simulink model "gm_FCS_MPC_3Phase_SPMSM_V1"  (R2022a)
settings: Solver=ode23t  StartTime=0.0  StopTime=0.2  RelTol=1e-3  AbsTol=1e-3  EnableMultiTasking=on
undefined symbols (not defined in the file or in its folder): f_c, Ld, Lq, np, psiPM, R, T_50MHz, u_dc
libraries: hdlmdlgenlib x28, dspsigops x26, ee_lib x22, nesl_utility x22, fl_lib x21, simulink x7
(part 2 of 5)

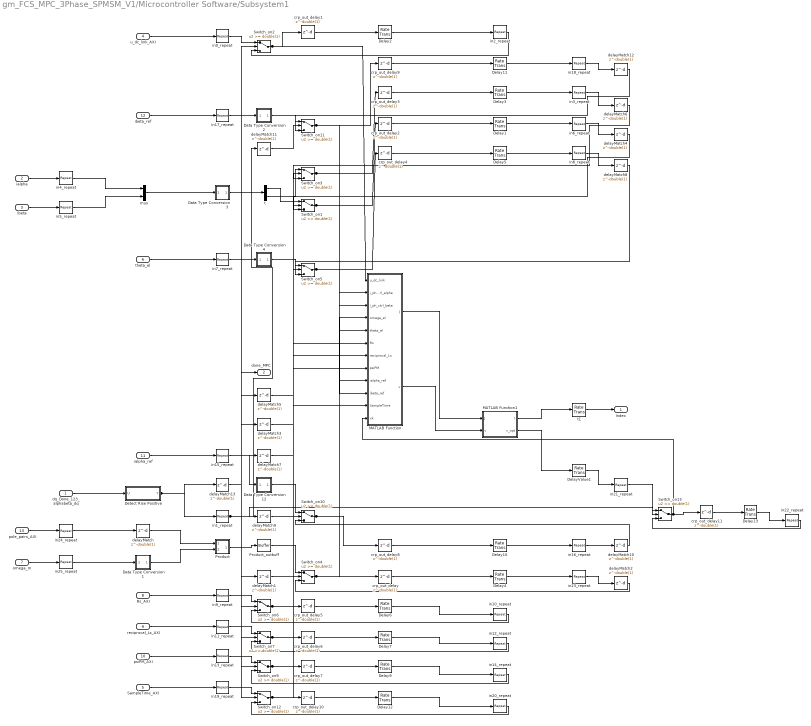
== system gm_FCS_MPC_3Phase_SPMSM_V1/Microcontroller Software/Subsystem1 ==
  dq_Done_123_alphabeta_dq : Inport  OutDataTypeStr=boolean  PortDimensions=1  SampleTime=1e-08
  ialpha : Inport  Port=2  OutDataTypeStr=fixdt(1, 18, 11)  PortDimensions=1  SampleTime=1e-08
  ibeta : Inport  Port=3  OutDataTypeStr=fixdt(1, 18, 11)  PortDimensions=1  SampleTime=1e-08
  u_dc_link_AXI : Inport  Port=4  OutDataTypeStr=single  PortDimensions=1  SampleTime=1e-08
  SampleTime_AXI : Inport  Port=5  OutDataTypeStr=single  PortDimensions=1  SampleTime=1e-08
  theta_el : Inport  Port=6  OutDataTypeStr=fixdt(1, 24, 20)  PortDimensions=1  SampleTime=1e-08
  omega_m : Inport  Port=7  OutDataTypeStr=fixdt(1, 24, 11)  PortDimensions=1  SampleTime=1e-08
  Rs_AXI : Inport  Port=8  OutDataTypeStr=single  PortDimensions=1  SampleTime=1e-08
  reciprocal_Ls_AXI : Inport  Port=9  OutDataTypeStr=single  PortDimensions=1  SampleTime=1e-08
  psiPM_AXI : Inport  Port=10  OutDataTypeStr=single  PortDimensions=1  SampleTime=1e-08
  ialpha_ref : Inport  Port=11  OutDataTypeStr=fixdt(1, 18, 11)  PortDimensions=1  SampleTime=1e-08
  ibeta_ref : Inport  Port=12  OutDataTypeStr=fixdt(1, 18, 11)  PortDimensions=1  SampleTime=1e-08
  pole_pairs_AXI : Inport  Port=13  OutDataTypeStr=single  PortDimensions=1  SampleTime=1e-08
  Data Type Conversion1 : Subsystem
      mask Display: disp('NFP\nconv');
  Data Type Conversion12 : Subsystem
      mask Display: disp('NFP\nconv');
  Data Type Conversion2 : Subsystem
      mask Display: disp('NFP\nconv');
  Data Type Conversion3 : Subsystem
      mask Display: disp('NFP\nconv');
  Data Type Conversion4 : Subsystem
      mask Display: disp('NFP\nconv');
  Delay{1..7,9..13} (12 alike) : RateTransition  OutPortSampleTimeOpt=Multiple of input port sample time  OutPortSampleTimeMultiple=100
  DelayValue1 : RateTransition  OutPortSampleTimeOpt=Multiple of input port sample time  OutPortSampleTimeMultiple=100
  Detect Rise Positive : Subsystem  mask(Detect Rise Positive){vinit=double(0), InputProcessing=Elements as channels (sample based), OutDataTypeStr=boolean}
      mask prompts: vinit "Simulink:masks:InitialCondition_MP"; InputProcessing "Simulink:masks:InputProcessing_MP"; OutDataTypeStr "Simulink:masks:OutputDataType_MP"
      mask help: Simulink:masks:DetectRisePositive_MD
      mask TypeOptions InputProcessing: Simulink:masks:ColumnsAsChannelsFrameBased | Simulink:masks:ElementsAsChannelsSampleBased
      mask TypeOptions OutDataTypeStr: Simulink:masks:uint8 | Simulink:masks:boolean
      mask Display: fprintf('U > 0\n&  NOT\nU/z > 0')
  MATLAB Function : Subsystem
  MATLAB Function1 : Subsystem
  Product : Subsystem
      mask Display: disp('NFP\nmul');
  Product_outbuff : hdlmdlgenlib/Buffer
      settings: SourceProductBaseCode=SL
  Switch_on{1..7,9..13} (12 alike) : Switch  Threshold=double(1)  OutDataTypeStr=single  RndMeth=Simplest  SampleTime=1e-10  SaturateOnIntegerOverflow=off  InputSameDT=off
  crp_out_delay{,1..11} (12 alike) : Delay  DelayLength=double(1)  InitialCondition=0  SampleTime=1e-10
  delayMatch{,1..12} (13 alike) : Delay  DelayLength=double(1)  InitialCondition=0  SampleTime=1e-10
  delayMatch13 : Delay  DelayLength=double(1)  InitialCondition=0  SampleTime=1e-08
  in0_repeat : dspsigops/Repeat  N=double(100)  RateOptions=Allow multirate processing  ic=0  mode=Unused parameter value
  in10_repeat : dspsigops/Repeat  N=double(100)  RateOptions=Allow multirate processing  ic=0  mode=Unused parameter value
  in11_repeat : dspsigops/Repeat  N=double(100)  RateOptions=Allow multirate processing  ic=0  mode=Unused parameter value
  in12_repeat : dspsigops/Repeat  N=double(100)  RateOptions=Allow multirate processing  ic=0  mode=Unused parameter value
  in13_repeat : dspsigops/Repeat  N=double(100)  RateOptions=Allow multirate processing  ic=0  mode=Unused parameter value
  in14_repeat : dspsigops/Repeat  N=double(100)  RateOptions=Allow multirate processing  ic=0  mode=Unused parameter value
  in15_repeat : dspsigops/Repeat  N=double(100)  RateOptions=Allow multirate processing  ic=0  mode=Unused parameter value
  in16_repeat : dspsigops/Repeat  N=double(100)  RateOptions=Allow multirate processing  ic=0  mode=Unused parameter value
  in17_repeat : dspsigops/Repeat  N=double(100)  RateOptions=Allow multirate processing  ic=0  mode=Unused parameter value
  in18_repeat : dspsigops/Repeat  N=double(100)  RateOptions=Allow multirate processing  ic=0  mode=Unused parameter value
  in19_repeat : dspsigops/Repeat  N=double(100)  RateOptions=Allow multirate processing  ic=0  mode=Unused parameter value
  in1_repeat : dspsigops/Repeat  N=double(100)  RateOptions=Allow multirate processing  ic=0  mode=Unused parameter value
  in20_repeat : dspsigops/Repeat  N=double(100)  RateOptions=Allow multirate processing  ic=0  mode=Unused parameter value
  in21_repeat : dspsigops/Repeat  N=double(100)  RateOptions=Allow multirate processing  ic=0  mode=Unused parameter value
  in22_repeat : dspsigops/Repeat  N=double(100)  RateOptions=Allow multirate processing  ic=0  mode=Unused parameter value
  in23_repeat : dspsigops/Repeat  N=double(100)  RateOptions=Allow multirate processing  ic=0  mode=Unused parameter value
  in24_repeat : dspsigops/Repeat  N=double(100)  RateOptions=Allow multirate processing  ic=0  mode=Unused parameter value
  in25_repeat : dspsigops/Repeat  N=double(100)  RateOptions=Allow multirate processing  ic=0  mode=Unused parameter value
  in2_repeat : dspsigops/Repeat  N=double(100)  RateOptions=Allow multirate processing  ic=0  mode=Unused parameter value
  in3_repeat : dspsigops/Repeat  N=double(100)  RateOptions=Allow multirate processing  ic=0  mode=Unused parameter value
  in4_repeat : dspsigops/Repeat  N=double(100)  RateOptions=Allow multirate processing  ic=0  mode=Unused parameter value
  in5_repeat : dspsigops/Repeat  N=double(100)  RateOptions=Allow multirate processing  ic=0  mode=Unused parameter value
  in6_repeat : dspsigops/Repeat  N=double(100)  RateOptions=Allow multirate processing  ic=0  mode=Unused parameter value
  in7_repeat : dspsigops/Repeat  N=double(100)  RateOptions=Allow multirate processing  ic=0  mode=Unused parameter value
  in8_repeat : dspsigops/Repeat  N=double(100)  RateOptions=Allow multirate processing  ic=0  mode=Unused parameter value
  in9_repeat : dspsigops/Repeat  N=double(100)  RateOptions=Allow multirate processing  ic=0  mode=Unused parameter value
  mux : Mux  Inputs=2
  t : Demux  Outputs=2
  t1 : RateTransition  OutPortSampleTimeOpt=Multiple of input port sample time  OutPortSampleTimeMultiple=100
  Index : Outport  SampleTime=1e-08
  done_MPC : Outport  Port=2  SampleTime=1e-08
  wires:
  dq_Done_123_alphabeta_dq/1 -> Detect Rise Positive/1(U)
  ialpha/1 -> in4_repeat/1
  ibeta/1 -> in5_repeat/1
  u_dc_link_AXI/1 -> in0_repeat/1
  SampleTime_AXI/1 -> in19_repeat/1
  theta_el/1 -> in7_repeat/1
  omega_m/1 -> in25_repeat/1
  Rs_AXI/1 -> in9_repeat/1
  reciprocal_Ls_AXI/1 -> in11_repeat/1
  psiPM_AXI/1 -> in13_repeat/1
  ialpha_ref/1 -> in15_repeat/1
  ibeta_ref/1 -> in17_repeat/1
  pole_pairs_AXI/1 -> in24_repeat/1
  delayMatch13/1 -> done_MPC/1
  t1/1 -> Index/1
  Detect Rise Positive/1(Y) -> delayMatch13/1, in1_repeat/1
  Delay4/1 -> in23_repeat/1
  DelayValue1/1 -> in21_repeat/1
  Delay2/1 -> in2_repeat/1
  Delay1/1 -> in6_repeat/1
  Delay3/1 -> in3_repeat/1
  Delay5/1 -> in8_repeat/1
  Delay6/1 -> in10_repeat/1
  Delay7/1 -> in12_repeat/1
  Delay9/1 -> in14_repeat/1
  Delay10/1 -> in16_repeat/1
  Delay11/1 -> in18_repeat/1
  Delay12/1 -> in20_repeat/1
  Delay13/1 -> in22_repeat/1
  in0_repeat/1 -> Switch_on2/1
  in1_repeat/1 -> delayMatch11/1, delayMatch9/1, delayMatch7/1, delayMatch5/1, delayMatch3/1, delayMatch1/1, Switch_on13/2, Switch_on12/2, Switch_on9/2, Switch_on7/2, Switch_on6/2, Switch_on2/2
  in2_repeat/1 -> Switch_on2/3
  in3_repeat/1 -> delayMatch6/1
  in4_repeat/1 -> mux/1
  in5_repeat/1 -> mux/2
  in6_repeat/1 -> delayMatch4/1
  in7_repeat/1 -> Data Type Conversion4/1(In1)
  in8_repeat/1 -> delayMatch8/1
  in9_repeat/1 -> Switch_on6/1
  in10_repeat/1 -> Switch_on6/3
  in11_repeat/1 -> Switch_on7/1
  in12_repeat/1 -> Switch_on7/3
  in13_repeat/1 -> Switch_on9/1
  in14_repeat/1 -> Switch_on9/3
  in15_repeat/1 -> Data Type Conversion12/1(In1)
  in16_repeat/1 -> delayMatch10/1
  in17_repeat/1 -> Data Type Conversion2/1(In1)
  in18_repeat/1 -> delayMatch12/1
  in19_repeat/1 -> Switch_on12/1
  in20_repeat/1 -> Switch_on12/3
  in21_repeat/1 -> Switch_on13/1
  in22_repeat/1 -> Switch_on13/3
  in23_repeat/1 -> delayMatch2/1
  in24_repeat/1 -> delayMatch/1
  in25_repeat/1 -> Data Type Conversion1/1(In1)
  crp_out_delay/1 -> Delay4/1
  MATLAB Function1/1(I) -> t1/1
  MATLAB Function1/2(v_opt) -> DelayValue1/1
  crp_out_delay1/1 -> Delay2/1
  crp_out_delay2/1 -> Delay1/1
  crp_out_delay3/1 -> Delay3/1
  crp_out_delay4/1 -> Delay5/1
  crp_out_delay5/1 -> Delay6/1
  crp_out_delay6/1 -> Delay7/1
  crp_out_delay7/1 -> Delay9/1
  crp_out_delay8/1 -> Delay10/1
  crp_out_delay9/1 -> Delay11/1
  crp_out_delay10/1 -> Delay12/1
  crp_out_delay11/1 -> Delay13/1
  Switch_on2/1 -> crp_out_delay1/1, MATLAB Function/1(u_dc_link)
  Switch_on3/1 -> crp_out_delay3/1, MATLAB Function/3(i_ph_ctrl_beta)
  mux/1 -> Data Type Conversion3/1(In1)
  Switch_on1/1 -> crp_out_delay2/1, MATLAB Function/2(i_ph_ctrl_alpha)
  Switch_on5/1 -> crp_out_delay4/1, MATLAB Function/5(theta_el)
  Switch_on6/1 -> crp_out_delay5/1, MATLAB Function/6(Rs)
  Switch_on7/1 -> crp_out_delay6/1, MATLAB Function/7(reciprocal_Ls)
  Switch_on9/1 -> crp_out_delay7/1, MATLAB Function/8(psiPM)
  Switch_on10/1 -> crp_out_delay8/1, MATLAB Function/9(ialpha_ref)
  Switch_on11/1 -> crp_out_delay9/1, MATLAB Function/10(ibeta_ref)
  Switch_on12/1 -> crp_out_delay10/1, MATLAB Function/11(SampleTime)
  Switch_on13/1 -> crp_out_delay11/1, MATLAB Function/12(vk)
  MATLAB Function/1(J) -> MATLAB Function1/1(J)
  MATLAB Function/2(v) -> MATLAB Function1/2(v)
  Switch_on4/1 -> crp_out_delay/1, MATLAB Function/4(omega_el)
  Product_outbuff/1 -> Switch_on4/1
  t/1 -> Switch_on1/1
  t/2 -> Switch_on3/1
  delayMatch1/1 -> Switch_on4/2
  delayMatch6/1 -> Switch_on3/3
  delayMatch4/1 -> Switch_on1/3
  delayMatch8/1 -> Switch_on5/3
  delayMatch10/1 -> Switch_on10/3
  delayMatch12/1 -> Switch_on11/3
  delayMatch2/1 -> Switch_on4/3
  delayMatch/1 -> Product/1(In1)
  Data Type Conversion3/1(Out1) -> t/1
  Data Type Conversion4/1(Out1) -> Switch_on5/1
  Data Type Conversion12/1(Out1) -> Switch_on10/1
  Data Type Conversion2/1(Out1) -> Switch_on11/1
  Product/1(Out1) -> Product_outbuff/1
  Data Type Conversion1/1(Out1) -> Product/2(In2)
  delayMatch3/1 -> Switch_on1/2
  delayMatch5/1 -> Switch_on3/2
  delayMatch7/1 -> Switch_on5/2
  delayMatch9/1 -> Switch_on10/2
  delayMatch11/1 -> Switch_on11/2

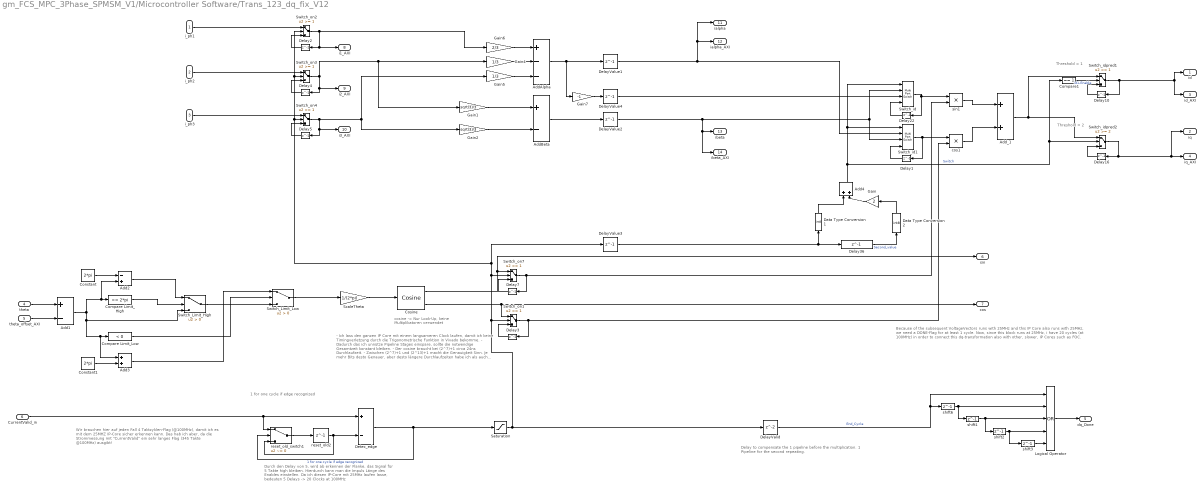
== system gm_FCS_MPC_3Phase_SPMSM_V1/Microcontroller Software/Trans_123_dq_fix_V12 ==
  note: Delay to compensate the 1 pipeline before the multiplication.
      | 1 Pipeline for the second repeating.
  note: cosine -> Nur Look-Up,
      | keine Multiplikatoren
      | verwendet
  note: - Ich lass den ganzen IP Core mit einem langsameren Clock laufen,
      | damit ich keine Timingverletzung durch die Trigonometrische
      | Funktion in Vivado bekomme.
      | - Dadurch das ich unnütze Pipeline Stages einspare, sollte
      | die notwendige Gesamtzeit konstant bleiben.
      | - Der cosine braucht bei (2^7)+1 circa 24ns Durchlaufzeit.
      | - Zwischen (2^7)+1 und (2^13)+1 macht die Genauigkeit Sinn. Je mehr Bits
      | desto Genauer, aber desto längere Durchlaufzeiten habe ich als auch mehr
      | Ressourcen brauche ich. (Habe mich aktuell für (2^9)+1 entschieden.
  note: Durch den Delay von 5, wird ab erkennen der Flanke,
      |  das Signal für 5 Takte high bleiben.
      | Hierdurch kann man die Impuls Länge des Enables einstellen.
      | Da ich diesen IP-Core mit 25MHz laufen lasse, bedeuten 5 Delays -> 20 Clocks at 100MHz
  note: 1 for one cycle if edge recognized
  note: Wir brauchen hier auf jeden Fall 4 Taktzyklen-Flag (@100MHz),
      | damit ich es mit dem 25MHZ IP-Core sicher erkennen kann. Das hab
      | ich aber, da die Strommessung mit "CurrentValid" ein sehr langes Flag
      | (345 Takte @100MHz) ausgibt!
  note: Because of the subsequent VoltageVectors runs with 25MHz and this
      | IP Core also runs with 25MHz, we need a DONE-Flag for at least 1 cycle.
      | Now, since this block runs at 25MHz, i have 20 cycles (at 100MHz) in order
      | to connect this dq-transformation also with other, slower, IP Cores such as
      | FOC.
  note: Threshold = 1
  note: Threshold = 2
  i_ph1 : Inport
  i_ph2 : Inport  Port=2
  i_ph3 : Inport  Port=3
  theta : Inport  Port=4
  theta_offset_AXI : Inport  Port=5
  CurrentValid_in : Inport  Port=6
  Add1 : Sum  Inputs=+-  OutDataTypeStr=Inherit: Same as accumulator
  Add2 : Sum  Inputs=-+  OutDataTypeStr=Inherit: Same as first input
  Add3 : Sum  OutDataTypeStr=Inherit: Same as first input
  Add4 : Sum  AccumDataTypeStr=int8  OutDataTypeStr=int8  RndMeth=Simplest
  AddAlpha : Sum  Inputs=+--  OutDataTypeStr=Inherit: Same as accumulator
  AddBeta : Sum  Inputs=+-  OutDataTypeStr=Inherit: Same as accumulator
  Add_1 : Sum  OutDataTypeStr=Inherit: Same as accumulator
  Compare Limit_High : simulink/Logic and Bit Operations/Compare To Constant  relop=>=  const=2*pi  OutDataTypeStr=boolean
  Compare Limit_Low : simulink/Logic and Bit Operations/Compare To Constant  relop=<  const=0  OutDataTypeStr=boolean
  Compare1 : simulink/Logic and Bit Operations/Compare To Constant  relop===  const=1  OutDataTypeStr=boolean
  Constant : Constant  Value=2*pi  OutDataTypeStr=fixdt(1,24,20)  SampleTime=T_50MHz
  Constant1 : Constant  Value=2*pi  OutDataTypeStr=fixdt(1,24,20)  SampleTime=T_50MHz
  Cosine : simulink/Lookup Tables/Cosine  Formula=sin(2*pi*u) and cos(2*pi*u)  NumDataPoints=(2^9)+1  OutputWordLength=16  InternalRulePriority=Precision
      settings: SourceProductBaseCode=SL
  Data Type Conversion1 : DataTypeConversion  OutDataTypeStr=int8  SaturateOnIntegerOverflow=off  RndMeth=Floor
  Data Type Conversion2 : DataTypeConversion  OutDataTypeStr=int8  SaturateOnIntegerOverflow=off  RndMeth=Floor
  Delay{1..5,7,10,16,22,36} (10 alike) : Delay  DelayLength=1
  DelayValid : Delay
  DelayValue{1..4} (4 alike) : Delay  DelayLength=1
  Detec_edge : Sum  Inputs=+-  AccumDataTypeStr=int8  OutDataTypeStr=int8
  Gain : Gain  Gain=2  RndMeth=Simplest
  Gain1 : Gain  Gain=sqrt(3)/3  OutDataTypeStr=Inherit: Same as input
  Gain2 : Gain  Gain=sqrt(3)/3  OutDataTypeStr=Inherit: Same as input
  Gain4 : Gain  Gain=1/3  OutDataTypeStr=Inherit: Same as input
  Gain5 : Gain  Gain=1/3  OutDataTypeStr=Inherit: Same as input
  Gain6 : Gain  Gain=2/3  OutDataTypeStr=Inherit: Same as input
  Gain7 : Gain  Gain=-1  OutDataTypeStr=Inherit: Same as input
  Logical Operator : Logic  Operator=OR  Inputs=5  AllPortsSameDT=off  OutDataTypeStr=boolean
  Saturation : Saturate  UpperLimit=1  LowerLimit=0  OutMin=[0]  OutMax=[1]  OutDataTypeStr=fixdt(0,1)
  ScaleTheta : Gain  Gain=1/(2*pi)  OutDataTypeStr=Inherit: Same as input
  Switch_Limit_High : Switch  Criteria=u2 > Threshold  OutDataTypeStr=fixdt(1,24,20)  SaturateOnIntegerOverflow=off  InputSameDT=off
  Switch_Limit_Low : Switch  Criteria=u2 > Threshold  OutDataTypeStr=fixdt(1,24,20)  SaturateOnIntegerOverflow=off  InputSameDT=off
  Switch_id : MultiPortSwitch  Inputs=2  DataPortForDefault=Additional data port  DiagnosticForDefault=None  OutDataTypeStr=Inherit: Inherit via back propagation  RndMeth=Simplest  SaturateOnIntegerOverflow=off  InputSameDT=off
  Switch_id1 : MultiPortSwitch  Inputs=2  DataPortForDefault=Additional data port  DiagnosticForDefault=None  OutDataTypeStr=Inherit: Inherit via back propagation  RndMeth=Simplest  SaturateOnIntegerOverflow=off  InputSameDT=off
  Switch_idpred1 : Switch  Threshold=1  OutDataTypeStr=Inherit: Inherit via back propagation  RndMeth=Simplest  SaturateOnIntegerOverflow=off  InputSameDT=off
  Switch_idpred2 : Switch  Threshold=2  OutDataTypeStr=Inherit: Inherit via back propagation  RndMeth=Simplest  SaturateOnIntegerOverflow=off  InputSameDT=off
  Switch_on1 : Switch  Threshold=1  OutDataTypeStr=fixdt(1,16,14)  SaturateOnIntegerOverflow=off  InputSameDT=off
  Switch_on2 : Switch  Threshold=1  OutDataTypeStr=Inherit: Inherit via back propagation  RndMeth=Simplest  SaturateOnIntegerOverflow=off  InputSameDT=off
  Switch_on3 : Switch  Threshold=1  OutDataTypeStr=Inherit: Inherit via back propagation  RndMeth=Simplest  SaturateOnIntegerOverflow=off  InputSameDT=off
  Switch_on4 : Switch  Threshold=1  OutDataTypeStr=Inherit: Inherit via back propagation  RndMeth=Simplest  SaturateOnIntegerOverflow=off  InputSameDT=off
  Switch_on7 : Switch  Threshold=1  OutDataTypeStr=fixdt(1,16,14)  SaturateOnIntegerOverflow=off  InputSameDT=off
  cos1 : Product  RndMeth=Simplest  OutDataTypeStr=Inherit: Same as first input
  reset_old2 : Delay  DelayLength=1
  reset_old_switch1 : Switch  Criteria=u2 ~= 0  SaturateOnIntegerOverflow=off  InputSameDT=off
  shift{1..3,6} (4 alike) : Delay  DelayLength=1
  sin1 : Product  RndMeth=Simplest  OutDataTypeStr=Inherit: Same as first input
  id : Outport  VectorParamsAs1DForOutWhenUnconnected=off
  iq : Outport  Port=2  VectorParamsAs1DForOutWhenUnconnected=off
  id_AXI : Outport  Port=3  VectorParamsAs1DForOutWhenUnconnected=off
  iq_AXI : Outport  Port=4  VectorParamsAs1DForOutWhenUnconnected=off
  dq_Done : Outport  Port=5  VectorParamsAs1DForOutWhenUnconnected=off
  sin : Outport  Port=6  VectorParamsAs1DForOutWhenUnconnected=off
  cos : Outport  Port=7  VectorParamsAs1DForOutWhenUnconnected=off
  i1_AXI : Outport  Port=8  VectorParamsAs1DForOutWhenUnconnected=off
  i2_AXI : Outport  Port=9  VectorParamsAs1DForOutWhenUnconnected=off
  i3_AXI : Outport  Port=10  VectorParamsAs1DForOutWhenUnconnected=off
  ialpha : Outport  Port=11  VectorParamsAs1DForOutWhenUnconnected=off
  ialpha_AXI : Outport  Port=12  VectorParamsAs1DForOutWhenUnconnected=off
  ibeta : Outport  Port=13  VectorParamsAs1DForOutWhenUnconnected=off
  ibeta_AXI : Outport  Port=14  VectorParamsAs1DForOutWhenUnconnected=off
  wires:
  Gain1/1 -> AddBeta/1
  Gain2/1 -> AddBeta/2
  theta/1 -> Add1/1
  Add1/1 -> Switch_Limit_High/3, Add3/1, Compare Limit_Low/1, Add2/2, Compare Limit_High/1
  theta_offset_AXI/1 -> Add1/2
  Switch_Limit_High/1 -> Switch_Limit_Low/3
  Compare Limit_High/1 -> Switch_Limit_High/2
  Compare Limit_Low/1 -> Switch_Limit_Low/2
  Constant/1 -> Add2/1
  Add2/1 -> Switch_Limit_High/1
  Constant1/1 -> Add3/2
  Add3/1 -> Switch_Limit_Low/1
  Switch_idpred2/1 -> iq/1, iq_AXI/1, Delay16/1
  Switch_idpred1/1 -> Delay10/1, id/1, id_AXI/1
  Saturation/1 -> DelayValid/1, Switch_on1/2, Switch_on7/2, DelayValue3/1, Switch_on2/2, Switch_on3/2, Switch_on4/2
  Delay3/1 -> Switch_on1/3
  Delay7/1 -> Switch_on7/3
  ScaleTheta/1 -> Cosine/1
  Cosine/2 -> cos/1, Switch_on1/1
  Switch_on7/1 -> Delay7/1, sin1/2
  Cosine/1 -> sin/1, Switch_on7/1
  Switch_on1/1 -> Delay3/1, cos1/2
  Switch_Limit_Low/1 -> ScaleTheta/1
  Gain4/1 -> AddAlpha/2
  Gain5/1 -> AddAlpha/3
  Gain6/1 -> AddAlpha/1
  Detec_edge/1 -> Saturation/1, reset_old_switch1/2  "1 for one cycle if edge recognized"
  reset_old2/1 -> reset_old_switch1/3, Detec_edge/2
  CurrentValid_in/1 -> reset_old_switch1/1, Detec_edge/1
  reset_old_switch1/1 -> reset_old2/1
  Delay2/1 -> Switch_on2/3
  Switch_on2/1 -> Delay2/1, i1_AXI/1, Gain6/1
  i_ph1/1 -> Switch_on2/1
  Switch_on3/1 -> i2_AXI/1, Delay4/1, Gain1/1, Gain4/1
  Delay4/1 -> Switch_on3/3
  i_ph2/1 -> Switch_on3/1
  Switch_on4/1 -> i3_AXI/1, Delay5/1, Gain2/1, Gain5/1
  Delay5/1 -> Switch_on4/3
  i_ph3/1 -> Switch_on4/1
  AddAlpha/1 -> Gain7/1, DelayValue1/1
  AddBeta/1 -> DelayValue2/1
  DelayValid/1 -> shift6/1, Logical Operator/1  "End_Cycle"
  shift6/1 -> Logical Operator/2, shift1/1
  Logical Operator/1 -> dq_Done/1
  Delay10/1 -> Switch_idpred1/3
  Delay16/1 -> Switch_idpred2/3
  Compare1/1 -> Switch_idpred1/2  "id1-Enable"
  Delay22/1 -> Switch_id/4
  Add4/1 -> Switch_idpred2/2, Compare1/1, Switch_id1/1, Switch_id/1  "Switch"
  sin1/1 -> Add_1/1
  cos1/1 -> Add_1/2
  DelayValue1/1 -> ialpha/1, ialpha_AXI/1, Switch_id1/2
  Switch_id/1 -> sin1/1, Delay22/1
  Delay1/1 -> Switch_id1/4
  Switch_id1/1 -> cos1/1, Delay1/1
  DelayValue3/1 -> Data Type Conversion1/1, Delay36/1
  Data Type Conversion1/1 -> Add4/1
  Gain/1 -> Add4/2
  Delay36/1 -> Data Type Conversion2/1  "Second_value"
  Data Type Conversion2/1 -> Gain/1
  DelayValue2/1 -> ibeta_AXI/1, ibeta/1, Switch_id/2, Switch_id1/3
  Add_1/1 -> Switch_idpred1/1, Switch_idpred2/1
  DelayValue4/1 -> Switch_id/3
  Gain7/1 -> DelayValue4/1
  shift1/1 -> Logical Operator/3, shift2/1
  shift2/1 -> shift3/1, Logical Operator/4
  shift3/1 -> Logical Operator/5

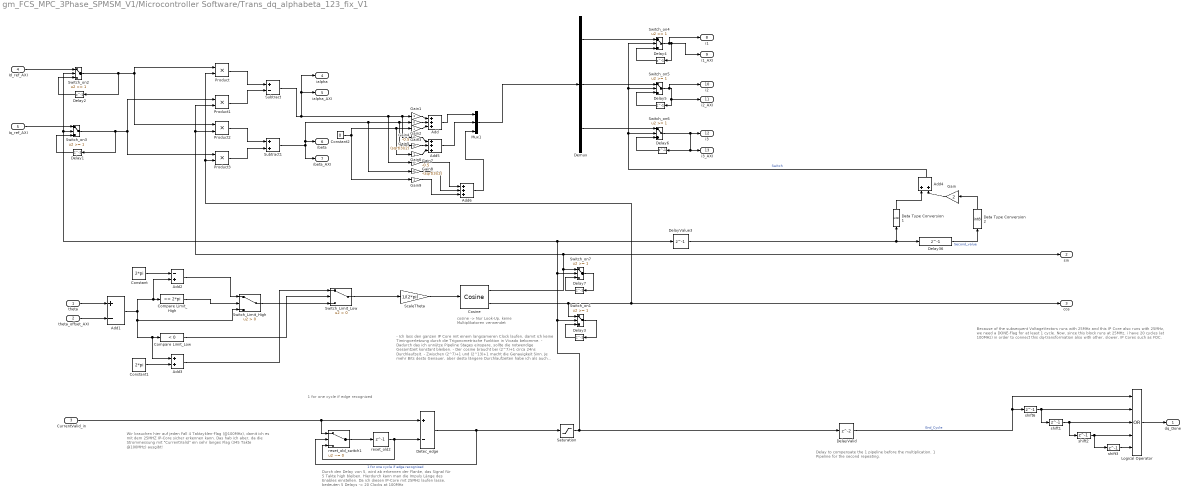
== system gm_FCS_MPC_3Phase_SPMSM_V1/Microcontroller Software/Trans_dq_alphabeta_123_fix_V1 ==
  note: Delay to compensate the 1 pipeline before the multiplication.
      | 1 Pipeline for the second repeating.
  note: cosine -> Nur Look-Up,
      | keine Multiplikatoren
      | verwendet
  note: - Ich lass den ganzen IP Core mit einem langsameren Clock laufen,
      | damit ich keine Timingverletzung durch die Trigonometrische
      | Funktion in Vivado bekomme.
      | - Dadurch das ich unnütze Pipeline Stages einspare, sollte
      | die notwendige Gesamtzeit konstant bleiben.
      | - Der cosine braucht bei (2^7)+1 circa 24ns Durchlaufzeit.
      | - Zwischen (2^7)+1 und (2^13)+1 macht die Genauigkeit Sinn. Je mehr Bits
      | desto Genauer, aber desto längere Durchlaufzeiten habe ich als auch mehr
      | Ressourcen brauche ich. (Habe mich aktuell für (2^9)+1 entschieden.
  note: Durch den Delay von 5, wird ab erkennen der Flanke,
      |  das Signal für 5 Takte high bleiben.
      | Hierdurch kann man die Impuls Länge des Enables einstellen.
      | Da ich diesen IP-Core mit 25MHz laufen lasse, bedeuten 5 Delays -> 20 Clocks at 100MHz
  note: 1 for one cycle if edge recognized
  note: Wir brauchen hier auf jeden Fall 4 Taktzyklen-Flag (@100MHz),
      | damit ich es mit dem 25MHZ IP-Core sicher erkennen kann. Das hab
      | ich aber, da die Strommessung mit "CurrentValid" ein sehr langes Flag
      | (345 Takte @100MHz) ausgibt!
  note: Because of the subsequent VoltageVectors runs with 25MHz and this
      | IP Core also runs with 25MHz, we need a DONE-Flag for at least 1 cycle.
      | Now, since this block runs at 25MHz, i have 20 cycles (at 100MHz) in order
      | to connect this dq-transformation also with other, slower, IP Cores such as
      | FOC.
  theta : Inport
  theta_offset_AXI : Inport  Port=2
  CurrentValid_in : Inport  Port=3
  Id_ref_AXI : Inport  Port=4
  Iq_ref_AXI : Inport  Port=5
  Add : Sum  Inputs=+++  OutDataTypeStr=fixdt(1,18,11)
  Add1 : Sum  Inputs=+-  OutDataTypeStr=Inherit: Same as accumulator
  Add2 : Sum  Inputs=-+  OutDataTypeStr=Inherit: Same as first input
  Add3 : Sum  OutDataTypeStr=Inherit: Same as first input
  Add4 : Sum  AccumDataTypeStr=int8  OutDataTypeStr=int8  RndMeth=Simplest
  Add5 : Sum  Inputs=+++  OutDataTypeStr=fixdt(1,18,11)
  Add6 : Sum  Inputs=+++  OutDataTypeStr=fixdt(1,18,11)
  Compare Limit_High : simulink/Logic and Bit Operations/Compare To Constant  relop=>=  const=2*pi  OutDataTypeStr=boolean
  Compare Limit_Low : simulink/Logic and Bit Operations/Compare To Constant  relop=<  const=0  OutDataTypeStr=boolean
  Constant : Constant  Value=2*pi  OutDataTypeStr=fixdt(1,24,20)  SampleTime=T_50MHz
  Constant1 : Constant  Value=2*pi  OutDataTypeStr=fixdt(1,24,20)  SampleTime=T_50MHz
  Constant2 : Constant  Value=0  OutDataTypeStr=fixdt(1,18,11)  SampleTime=-1
  Cosine : simulink/Lookup Tables/Cosine  Formula=sin(2*pi*u) and cos(2*pi*u)  NumDataPoints=(2^9)+1  OutputWordLength=16  InternalRulePriority=Precision
      settings: SourceProductBaseCode=SL
  Data Type Conversion1 : DataTypeConversion  OutDataTypeStr=int8  SaturateOnIntegerOverflow=off  RndMeth=Floor
  Data Type Conversion2 : DataTypeConversion  OutDataTypeStr=int8  SaturateOnIntegerOverflow=off  RndMeth=Floor
  Delay{1..7,36} (8 alike) : Delay  DelayLength=1
  DelayValid : Delay
  DelayValue3 : Delay  DelayLength=1
  Demux : Demux  Outputs=3
  Detec_edge : Sum  Inputs=+-  AccumDataTypeStr=int8  OutDataTypeStr=int8
  Gain : Gain  Gain=2  RndMeth=Simplest
  Gain{1,3,6,9} (4 alike) : Gain  OutDataTypeStr=fixdt(1,18,11)
  Gain2 : Gain  Gain=0  OutDataTypeStr=fixdt(1,18,11)
  Gain4 : Gain  Gain=-0.5  OutDataTypeStr=fixdt(1,18,11)
  Gain5 : Gain  Gain=(sqrt(3)/2)  OutDataTypeStr=fixdt(1,18,11)
  Gain7 : Gain  Gain=-0.5  OutDataTypeStr=fixdt(1,18,11)
  Gain8 : Gain  Gain=-(sqrt(3)/2)  OutDataTypeStr=fixdt(1,18,11)
  Logical Operator : Logic  Operator=OR  Inputs=5  AllPortsSameDT=off  OutDataTypeStr=boolean
  Mux1 : Mux  Inputs=3
  Product{,1..3} (4 alike) : Product  OutDataTypeStr=fixdt(1,18,11)
  Saturation : Saturate  UpperLimit=1  LowerLimit=0  OutMin=[0]  OutMax=[1]  OutDataTypeStr=fixdt(0,1)
  ScaleTheta : Gain  Gain=1/(2*pi)  OutDataTypeStr=Inherit: Same as input
  Subtract : Sum  Inputs=+-  OutDataTypeStr=fixdt(1,18,11)
  Subtract1 : Sum  OutDataTypeStr=fixdt(1,18,11)
  Switch_Limit_High : Switch  Criteria=u2 > Threshold  OutDataTypeStr=fixdt(1,24,20)  SaturateOnIntegerOverflow=off  InputSameDT=off
  Switch_Limit_Low : Switch  Criteria=u2 > Threshold  OutDataTypeStr=fixdt(1,24,20)  SaturateOnIntegerOverflow=off  InputSameDT=off
  Switch_on1 : Switch  Threshold=1  OutDataTypeStr=fixdt(1,16,14)  SaturateOnIntegerOverflow=off  InputSameDT=off
  Switch_on{2..6} (5 alike) : Switch  Threshold=1  OutDataTypeStr=Inherit: Inherit via back propagation  RndMeth=Simplest  SaturateOnIntegerOverflow=off  InputSameDT=off
  Switch_on7 : Switch  Threshold=1  OutDataTypeStr=fixdt(1,16,14)  SaturateOnIntegerOverflow=off  InputSameDT=off
  reset_old2 : Delay  DelayLength=1
  reset_old_switch1 : Switch  Criteria=u2 ~= 0  SaturateOnIntegerOverflow=off  InputSameDT=off
  shift{1..3,6} (4 alike) : Delay  DelayLength=1
  dq_Done : Outport  VectorParamsAs1DForOutWhenUnconnected=off
  sin : Outport  Port=2  VectorParamsAs1DForOutWhenUnconnected=off
  cos : Outport  Port=3  VectorParamsAs1DForOutWhenUnconnected=off
  ialpha : Outport  Port=4  VectorParamsAs1DForOutWhenUnconnected=off
  ialpha_AXI : Outport  Port=5  VectorParamsAs1DForOutWhenUnconnected=off
  ibeta : Outport  Port=6  VectorParamsAs1DForOutWhenUnconnected=off
  ibeta_AXI : Outport  Port=7  VectorParamsAs1DForOutWhenUnconnected=off
  i1 : Outport  Port=8  VectorParamsAs1DForOutWhenUnconnected=off
  i1_AXI : Outport  Port=9  VectorParamsAs1DForOutWhenUnconnected=off
  i2 : Outport  Port=10  VectorParamsAs1DForOutWhenUnconnected=off
  i2_AXI : Outport  Port=11  VectorParamsAs1DForOutWhenUnconnected=off
  i3 : Outport  Port=12  VectorParamsAs1DForOutWhenUnconnected=off
  i3_AXI : Outport  Port=13  VectorParamsAs1DForOutWhenUnconnected=off
  wires:
  theta/1 -> Add1/1
  Add1/1 -> Add2/2, Compare Limit_High/1, Switch_Limit_High/3, Add3/1, Compare Limit_Low/1
  theta_offset_AXI/1 -> Add1/2
  Switch_Limit_High/1 -> Switch_Limit_Low/3
  Compare Limit_High/1 -> Switch_Limit_High/2
  Compare Limit_Low/1 -> Switch_Limit_Low/2
  Constant/1 -> Add2/1
  Add2/1 -> Switch_Limit_High/1
  Constant1/1 -> Add3/2
  Add3/1 -> Switch_Limit_Low/1
  Saturation/1 -> DelayValid/1, Switch_on1/2, Switch_on7/2, Switch_on2/2, Switch_on3/2, DelayValue3/1
  Delay3/1 -> Switch_on1/3
  Delay7/1 -> Switch_on7/3
  ScaleTheta/1 -> Cosine/1
  Switch_on7/1 -> Delay7/1
  Switch_on1/1 -> Delay3/1
  Detec_edge/1 -> Saturation/1, reset_old_switch1/2  "1 for one cycle if edge recognized"
  reset_old2/1 -> reset_old_switch1/3, Detec_edge/2
  CurrentValid_in/1 -> reset_old_switch1/1, Detec_edge/1
  reset_old_switch1/1 -> reset_old2/1
  DelayValid/1 -> shift6/1, Logical Operator/1  "End_Cycle"
  shift6/1 -> Logical Operator/2, shift1/1
  Logical Operator/1 -> dq_Done/1
  DelayValue3/1 -> Data Type Conversion1/1, Delay36/1
  Data Type Conversion1/1 -> Add4/1
  Gain/1 -> Add4/2
  Delay36/1 -> Data Type Conversion2/1  "Second_value"
  Data Type Conversion2/1 -> Gain/1
  shift1/1 -> Logical Operator/3, shift2/1
  shift2/1 -> shift3/1, Logical Operator/4
  shift3/1 -> Logical Operator/5
  Id_ref_AXI/1 -> Switch_on2/1
  Delay2/1 -> Switch_on2/3
  Delay1/1 -> Switch_on3/3
  Iq_ref_AXI/1 -> Switch_on3/1
  Constant2/1 -> Gain9/1, Gain6/1, Gain3/1
  Demux/1 -> Switch_on4/1
  Switch_on4/1 -> i1_AXI/1, Delay4/1, i1/1
  Delay4/1 -> Switch_on4/3
  Delay5/1 -> Switch_on5/3
  Switch_on5/1 -> i2/1, i2_AXI/1, Delay5/1
  Demux/2 -> Switch_on5/1
  Delay6/1 -> Switch_on6/3
  Switch_on6/1 -> i3/1, i3_AXI/1, Delay6/1
  Demux/3 -> Switch_on6/1
  Gain1/1 -> Add/1
  Gain2/1 -> Add/2
  Gain3/1 -> Add/3
  Add/1 -> Mux1/1
  Gain5/1 -> Add5/2
  Gain4/1 -> Add5/1
  Gain6/1 -> Add5/3
  Add5/1 -> Mux1/2
  Gain8/1 -> Add6/2
  Gain7/1 -> Add6/1
  Gain9/1 -> Add6/3
  Add6/1 -> Mux1/3
  Add4/1 -> Switch_on6/2, Switch_on5/2, Switch_on4/2  "Switch"
  Mux1/1 -> Demux/1
  Switch_Limit_Low/1 -> ScaleTheta/1
  Subtract/1 -> Gain7/1, Gain4/1, Gain1/1, ialpha/1, ialpha_AXI/1
  Subtract1/1 -> Gain8/1, Gain5/1, Gain2/1, ibeta/1, ibeta_AXI/1
  Product1/1 -> Subtract/2
  Product2/1 -> Subtract1/1
  Product/1 -> Subtract/1
  Switch_on3/1 -> Delay1/1, Product1/1, Product3/1
  Switch_on2/1 -> Delay2/1, Product/1, Product2/1
  Product3/1 -> Subtract1/2
  Cosine/1 -> sin/1, Product2/2, Product1/2, Switch_on7/1
  Cosine/2 -> cos/1, Product3/2, Product/2, Switch_on1/1

== system gm_FCS_MPC_3Phase_SPMSM_V1/Microcontroller Software/Subsystem1/Data Type Conversion1 ==
  In1 : Inport
  Data Type Conversion1 : DataTypeConversion  OutDataTypeStr=single  RndMeth=Nearest  SampleTime=1e-10  SaturateOnIntegerOverflow=off
  Data Type Conversion1_pd1 : Delay  DelayLength=6
  Out1 : Outport
  wires:
  In1/1 -> Data Type Conversion1/1
  Data Type Conversion1/1 -> Data Type Conversion1_pd1/1
  Data Type Conversion1_pd1/1 -> Out1/1

== system gm_FCS_MPC_3Phase_SPMSM_V1/Microcontroller Software/Subsystem1/Data Type Conversion12 ==
  In1 : Inport
  Data Type Conversion12 : DataTypeConversion  OutDataTypeStr=single  RndMeth=Nearest  SampleTime=1e-10  SaturateOnIntegerOverflow=off
  Data Type Conversion12_pd1 : Delay  DelayLength=6
  Out1 : Outport
  wires:
  In1/1 -> Data Type Conversion12/1
  Data Type Conversion12/1 -> Data Type Conversion12_pd1/1
  Data Type Conversion12_pd1/1 -> Out1/1

== system gm_FCS_MPC_3Phase_SPMSM_V1/Microcontroller Software/Subsystem1/Data Type Conversion2 ==
  In1 : Inport
  Data Type Conversion2 : DataTypeConversion  OutDataTypeStr=single  RndMeth=Nearest  SampleTime=1e-10  SaturateOnIntegerOverflow=off
  Data Type Conversion2_pd1 : Delay  DelayLength=6
  Out1 : Outport
  wires:
  In1/1 -> Data Type Conversion2/1
  Data Type Conversion2/1 -> Data Type Conversion2_pd1/1
  Data Type Conversion2_pd1/1 -> Out1/1

== system gm_FCS_MPC_3Phase_SPMSM_V1/Microcontroller Software/Subsystem1/Data Type Conversion3 ==
  In1 : Inport
  Data Type Conversion3 : DataTypeConversion  OutDataTypeStr=single  RndMeth=Nearest  SampleTime=1e-10  SaturateOnIntegerOverflow=off
  Data Type Conversion3_pd1 : Delay  DelayLength=6
  Out1 : Outport
  wires:
  In1/1 -> Data Type Conversion3/1
  Data Type Conversion3/1 -> Data Type Conversion3_pd1/1
  Data Type Conversion3_pd1/1 -> Out1/1

== system gm_FCS_MPC_3Phase_SPMSM_V1/Microcontroller Software/Subsystem1/Data Type Conversion4 ==
  In1 : Inport
  Data Type Conversion4 : DataTypeConversion  OutDataTypeStr=single  RndMeth=Nearest  SampleTime=1e-10  SaturateOnIntegerOverflow=off
  Data Type Conversion4_pd1 : Delay  DelayLength=6
  Out1 : Outport
  wires:
  In1/1 -> Data Type Conversion4/1
  Data Type Conversion4/1 -> Data Type Conversion4_pd1/1
  Data Type Conversion4_pd1/1 -> Out1/1

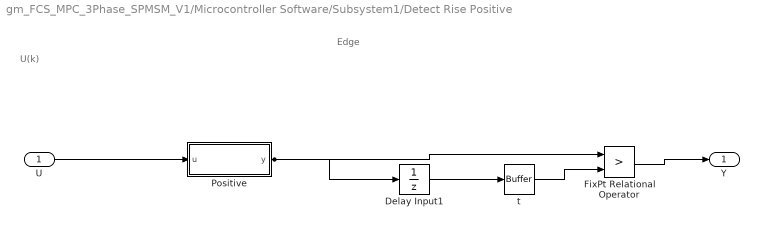
== system gm_FCS_MPC_3Phase_SPMSM_V1/Microcontroller Software/Subsystem1/Detect Rise Positive ==
  note: Edge
  note: U(k)
  U : Inport  OutDataTypeStr=boolean  SampleTime=1e-08
  Delay Input1 : UnitDelay  SampleTime=1e-08
  FixPt Relational Operator : RelationalOperator  Operator=>  OutDataTypeStr=boolean  SampleTime=1e-08  InputSameDT=off
  Positive : Subsystem  mask(Compare To Zero){relop=>, OutDataTypeStr=boolean, ZeroCross=off}
      mask prompts: relop "Simulink:masks:Operator_MP"; OutDataTypeStr "Simulink:masks:OutputDataType_MP"; ZeroCross "Simulink:masks:EnableZerocrossingDetection_MP"
      mask help: Simulink:masks:CompareToZero_MD
      mask TypeOptions relop: == | ~= | < | <= | >= | >
      mask TypeOptions OutDataTypeStr: Simulink:masks:uint8 | Simulink:masks:boolean
      mask Callback ZeroCross: sl('zeroCrossEnable', gcbh);
      mask Display: disp([relop,' 0'])
  t : hdlmdlgenlib/Buffer
      settings: SourceProductBaseCode=SL
  Y : Outport  SampleTime=1e-08
  wires:
  t/1 -> FixPt Relational Operator/2
  FixPt Relational Operator/1 -> Y/1
  Delay Input1/1 -> t/1
  Positive/1(y) -> FixPt Relational Operator/1, Delay Input1/1
  U/1 -> Positive/1(u)
